simulink model "FuncionesDeMembresiaDMA"  (R2025b)
settings: Solver=FixedStepAuto  StartTime=0.0  StopTime=10.0  FixedStep=0.001  RelTol=1e-3
values from neighbouring files (symbols this model uses):
  K_nl = squeeze(K(:,:,1))    [TakagiSugenoDMA.m]
  K_ns = squeeze(K(:,:,2))    [TakagiSugenoDMA.m]
  K_pl = squeeze(K(:,:,5))    [TakagiSugenoDMA.m]
  K_ps = squeeze(K(:,:,4))    [TakagiSugenoDMA.m]
  K_z = squeeze(K(:,:,3))    [TakagiSugenoDMA.m]
  W = 1    [TakagiSugenoDMA.m]
undefined symbols (not defined in the file or in its folder): G_nl, G_ns, G_pl, G_ps, G_z, P_nl, P_ns, P_pl, P_ps, P_z
settings Model: Creator=david  LastModifiedBy=david

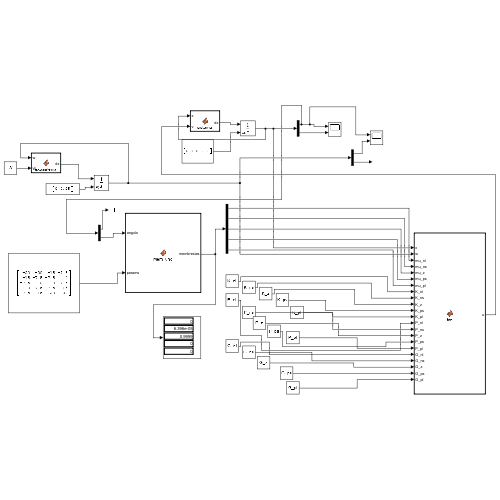
[thumbnail: Simulink's stored preview of the top-level diagram]
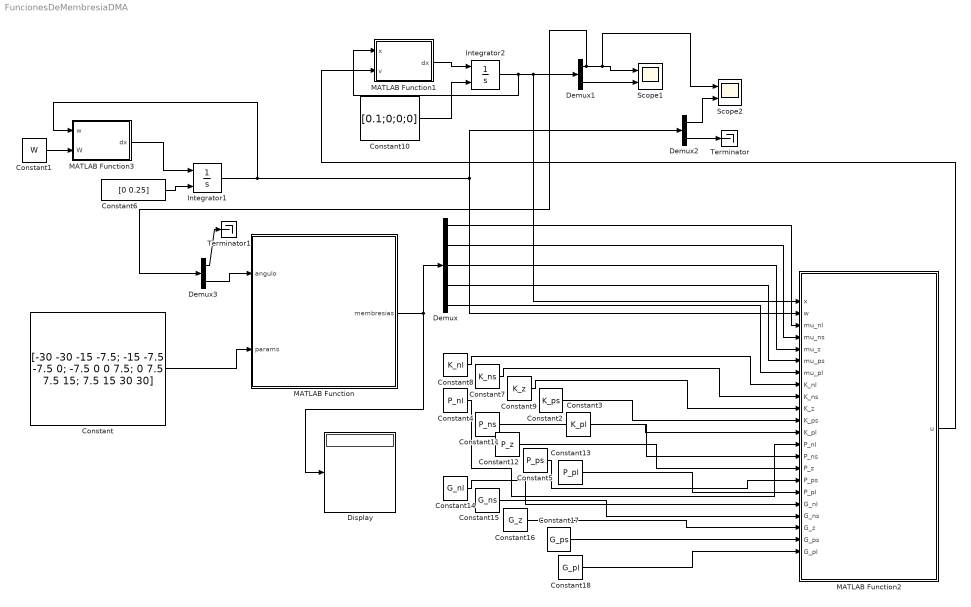
== system FuncionesDeMembresiaDMA ==
  Constant : Constant  Value=[-30 -30 -15 -7.5; -15 -7.5 -7.5 0; -7.5 0 0 7.5; 0 7.5 7.5 15; 7.5 15 30 30]
  Constant1 : Constant  Value=W
  Constant10 : Constant  Value=[0.1;0;0;0]
  Constant11 : Constant  Value=P_ns
  Constant12 : Constant  Value=P_z
  Constant13 : Constant  Value=P_pl
  Constant14 : Constant  Value=G_nl
  Constant15 : Constant  Value=G_ns
  Constant16 : Constant  Value=G_z
  Constant17 : Constant  Value=G_ps
  Constant18 : Constant  Value=G_pl
  Constant2 : Constant  Value=K_ps
  Constant3 : Constant  Value=K_pl
  Constant4 : Constant  Value=P_nl
  Constant5 : Constant  Value=P_ps
  Constant6 : Constant  Value=[0 0.25]
  Constant7 : Constant  Value=K_ns
  Constant8 : Constant  Value=K_nl
  Constant9 : Constant  Value=K_z
  Demux : Demux  Outputs=5
  Demux1 : Demux  Outputs=2
  Demux2 : Demux  Outputs=2
  Demux3 : Demux  Outputs=2
  Display : Display
  Integrator1 : Integrator  InitialConditionSource=external
  Integrator2 : Integrator  InitialConditionSource=external
  MATLAB Function : MATLAB Function  TreatAsAtomicUnit=on
  MATLAB Function1 : MATLAB Function  TreatAsAtomicUnit=on
  MATLAB Function2 : MATLAB Function  TreatAsAtomicUnit=on
  MATLAB Function3 : MATLAB Function  TreatAsAtomicUnit=on
  Scope1 : Scope  NumInputPorts=2
      settings: ActiveDisplayYMinimum=-3.2105  ActiveDisplayYMaximum=3.2105
  Scope2 : Scope  NumInputPorts=2
      settings: ActiveDisplayYMinimum=-0.36045772454197417  ActiveDisplayYMaximum=0.3646661600104299  DataLoggingVariableName=ScopeData2
  Terminator : Terminator
  Terminator1 : Terminator
  wires:
  Constant/1 -> MATLAB Function/2(params)
  MATLAB Function/1(membresias) -> Display/1, Demux/1
  Demux/5 -> MATLAB Function2/7(mu_pl)
  Demux/4 -> MATLAB Function2/6(mu_ps)
  Demux/3 -> MATLAB Function2/5(mu_z)
  Demux/2 -> MATLAB Function2/4(mu_ns)
  Demux/1 -> MATLAB Function2/3(mu_nl)
  Constant6/1 -> Integrator1/2
  Integrator1/1 -> MATLAB Function3/1(w), Demux2/1, MATLAB Function2/2(w)
  MATLAB Function3/1(dx) -> Integrator1/1
  Constant8/1 -> MATLAB Function2/8(K_nl)
  Constant7/1 -> MATLAB Function2/9(K_ns)
  Constant9/1 -> MATLAB Function2/10(K_z)
  MATLAB Function1/1(dx) -> Integrator2/1
  Constant10/1 -> Integrator2/2
  Integrator2/1 -> MATLAB Function2/1(x), Demux1/1, MATLAB Function1/1(x)
  Demux1/2 -> Scope1/2
  MATLAB Function2/1(u) -> MATLAB Function1/2(v)
  Demux2/2 -> Terminator/1
  Demux2/1 -> Scope2/2
  Demux1/1 -> Demux3/1, Scope2/1, Scope1/1
  Constant1/1 -> MATLAB Function3/2(W)
  Constant2/1 -> MATLAB Function2/11(K_ps)
  Constant3/1 -> MATLAB Function2/12(K_pl)
  Constant4/1 -> MATLAB Function2/13(P_nl)
  Constant11/1 -> MATLAB Function2/14(P_ns)
  Constant12/1 -> MATLAB Function2/15(P_z)
  Constant5/1 -> MATLAB Function2/16(P_ps)
  Constant13/1 -> MATLAB Function2/17(P_pl)
  Constant14/1 -> MATLAB Function2/18(G_nl)
  Constant15/1 -> MATLAB Function2/19(G_ns)
  Constant16/1 -> MATLAB Function2/20(G_z)
  Constant17/1 -> MATLAB Function2/21(G_ps)
  Constant18/1 -> MATLAB Function2/22(G_pl)
  Demux3/1 -> Terminator1/1
  Demux3/2 -> MATLAB Function/1(angulo)

== matlab function FuncionesDeMembresiaDMA/MATLAB Function1 ==
  data: x input; v input; dx output
function dx = sistema(x, v)
%#codegen

dx = zeros(4,1);   % asegura tamaño fijo 4x1

%% ---- Parámetros (paper) ----
m2 = 0.50;      % kg
l2 = 0.75;      % m
l1 = 0.12;      % m
J  = 0.003;     % kg*m^2
Km = 0.104;     % N*m/A
Kg = 0.055;     
Rm = 1.9;       % ohm
g  = 9.81;      % m/s^2

P1 = (Kg*Km)/Rm;
P2 = (Kg^2*Km^2)/Rm;

%% ---- Estados ----
th  = x(1);
al  = x(2);
dth = x(3);
dal = x(4);

%% ---- Dinámica ----
d11 = m2*l1^2 + J;
d12 = m2*l1*l2*cos(al);
d22 = m2*l2^2;
D = [d11 d12; d12 d22];

c12 = -m2*l1*l2*sin(al)*dal;
c21 =  m2*l1*l2*sin(al)*dth;
C = [0 c12; c21 0];

G = [0; m2*l2*g*sin(al)];

tau = P1*v - P2*dth;

qdot = [dth; dal];
rhs  = [tau] - C*qdot - G;
qdd  = D \ rhs;

dx = [dth; dal; qdd(1); qdd(2)];
end

== matlab function FuncionesDeMembresiaDMA/MATLAB Function ==
  data: angulo input; membresias output; params input
function membresias = MemFunc(angulo, params)
% calcular_membresia_flexible: Calcula los valores de membresía para un ángulo
%   dado usando una matriz de parámetros.
%   Input:
%       - angulo: El valor del ángulo (puede ser un escalar o un vector).
%       - params: Una matriz de M x N, donde M es el número de funciones
%                 de membresía y N es el número de parámetros por función.
%                 Formato esperado: [a, b, c, d] para trapezoidal o [a, b, c, c] para triangular.
%   Output:
%       - membresias: Un vector o matriz con los valores de membresía. Cada columna
%                     corresponde a una función de membresía.

% Obtener el número de funciones de membresía de la matriz de parámetros
num_funciones = size(params, 1);

% Inicializar la matriz de resultados. Si angulo es un vector, la matriz de
% resultados tendrá el mismo número de filas que angulo y el número de
% columnas de las funciones.
membresias = zeros(length(angulo), num_funciones);

% Recorrer cada función de membresía definida en la matriz de parámetros
for i = 1:num_funciones
    % Extraer los parámetros de la fila actual
    p = params(i, :);
    
    % Asignar los puntos de control. Si la matriz es 1x3, asumimos que es una triangular.
    if length(p) == 3
        a = p(1);
        b = p(2);
        c = p(3);
        d = p(3); % Para funciones triangulares, c y d son el mismo punto
    elseif length(p) == 4
        a = p(1);
        b = p(2);
        c = p(3);
        d = p(4);
    else
        error('La matriz de parámetros debe tener 3 o 4 columnas.');
    end
    
    % Calcular la membresía para cada ángulo de entrada usando la función 'trapmf'
    % de Fuzzy Logic Toolbox. Esta función puede manejar triángulos y trapezoides.
    % Si no tienes la toolbox, puedes implementar la fórmula manualmente como
    % en la respuesta anterior.
    
    % La siguiente es una implementación manual si no se tiene la toolbox
    mu = zeros(size(angulo));
    
    % Lado izquierdo del trapecio/triángulo
    idx1 = angulo > a & angulo <= b;
    mu(idx1) = (angulo(idx1) - a) / (b - a);
    
    % Parte superior del trapecio (valor 1)
    idx2 = angulo >= b & angulo <= c;
    mu(idx2) = 1;
    
    % Lado derecho del trapecio/triángulo
    idx3 = angulo > c & angulo < d;
    mu(idx3) = (d - angulo(idx3)) / (d - c);
    
    % Asignar el vector de membresía a la columna correspondiente
    membresias(:, i) = mu'; % Transponer si angulo es un vector fila
end

end

== matlab function FuncionesDeMembresiaDMA/MATLAB Function2 ==
  data: x input; u output; w input; mu_nl input; mu_ns input; mu_z input; mu_ps input; mu_pl input; K_nl input; K_ns input; K_z input; K_ps input; K_pl input; P_nl input; P_ns input; P_z input; P_ps input; P_pl input; G_nl input; G_ns input; G_z input; G_ps input; G_pl input
function u = fcn(x, w, mu_nl, mu_ns, mu_z, mu_ps, mu_pl, ...
                 K_nl, K_ns, K_z, K_ps, K_pl, ...
                 P_nl, P_ns, P_z, P_ps, P_pl, ...
                 G_nl, G_ns, G_z, G_ps, G_pl)

x    = x(:);        % asegura columna 4x1
K_nl = K_nl(:)';    % asegura fila 1x4
K_ns = K_ns(:)'; 
K_z  = K_z(:)'; 
K_ps = K_ps(:)'; 
K_pl = K_pl(:)'; 

%% Control local en cada punto TS
u_nl = -K_nl*x + (G_nl - K_nl*P_nl)*w;
u_ns = -K_ns*x + (G_ns - K_ns*P_ns)*w;
u_z  = -K_z *x + (G_z  - K_z *P_z )*w;
u_ps = -K_ps*x + (G_ps - K_ps*P_ps)*w;
u_pl = -K_pl*x + (G_pl - K_pl*P_pl)*w;

%% Combinación convexa
den = mu_nl + mu_ns + mu_z + mu_ps + mu_pl;
if den == 0
    u = zeros(size(u_nl));
else
    u = (u_nl*mu_nl + u_ns*mu_ns + u_z*mu_z + ...
         u_ps*mu_ps + u_pl*mu_pl) / den;
end

end

== matlab function FuncionesDeMembresiaDMA/MATLAB Function3 ==
  data: w input; dx output; W input
function dx = exosistema(w,W)
%#codegen
dx = zeros(2,1);        % asegura que Simulink sepa el tamaño
A  = [0 W; -W 0];
dx = A*w;
end
